simulink model "SRE_Integral"  (R2021a)
settings: Solver=VariableStepAuto  StartTime=0.0  StopTime=20.0  RelTol=1e-3
values from neighbouring files (symbols this model uses):
  G = ss(Ad, Bd, Cd, Dd, Ts)    [controlador_RE.m]    (also in realim_estados_no_ff.m)
  K = acker(A_ext, B_ext, exp(Ts*p_C))    [controlador_RE.m]    (also in realim_estados_no_ff.m = [0.2533,   -0.0121, -116.5175,  -30])
  L_o = [ 0.0003  0.0002 ... (first row only)    [controlador_RE.m]
  Ts = 20e-3    (= 0.02)    [controlador_RE.m]    (also in realim_estados_no_ff.m)
undefined symbols (not defined in the file or in its folder): DiscIntNeverNeededParam
libraries: simulink x1
settings Model: Creator=mathe  LastModifiedBy=mathe

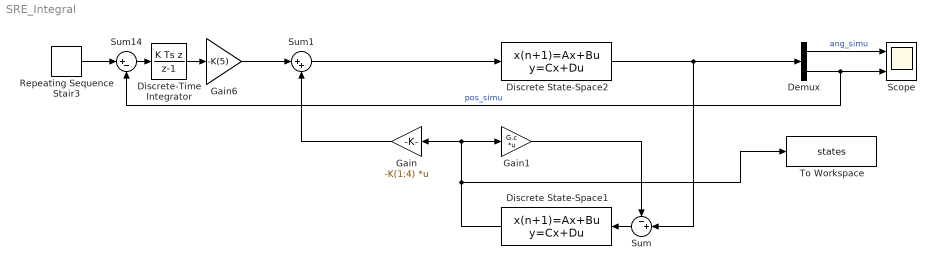
== system SRE_Integral ==
  Demux : Demux  Outputs=2
  Discrete State-Space1 : DiscreteStateSpace  A=G.a-G.b*K(1:4)  B=L_o  C=eye(4)  D=zeros(4,2)  InitialCondition=[0 0 0 0]  SampleTime=Ts
  Discrete State-Space2 : DiscreteStateSpace  A=G.a  B=G.b  C=G.c  D=zeros(2,1)  InitialCondition=[0 0 0 0]  SampleTime=Ts
  Discrete-Time Integrator : DiscreteIntegrator  IntegratorMethod=Integration: Backward Euler  SampleTime=-1  ICPrevOutput=DiscIntNeverNeededParam  ICPrevScaledInput=DiscIntNeverNeededParam
  Gain : Gain  Gain=-K(1:4)  Multiplication=Matrix(K*u)
  Gain1 : Gain  Gain=G.c  Multiplication=Matrix(K*u)
  Gain6 : Gain  Gain=-K(5)
  Repeating Sequence Stair3 : simulink/Sources/Repeating Sequence Stair  OutValues=[0 0.1 -.10].'  tsamp=5  OutMin=[]  OutMax=[]  OutDataTypeStr=double  OutputDataTypeScalingMode=double  OutDataType=fixdt(0,8)  ConRadixGroup=Best Precision: Vector-wise  OutScaling=2^-12
  Scope : Scope  NumInputPorts=2
  Sum : Sum  Inputs=-+|
  Sum1 : Sum  Inputs=|++
  Sum14 : Sum  Inputs=|+-
  To Workspace : ToWorkspace  VariableName=states  SampleTime=-1
      settings: Save2DSignal=2-D array (concatenate along first dimension)
  wires:
  Discrete State-Space1/1 -> To Workspace/1, Gain1/1, Gain/1
  Discrete State-Space2/1 -> Sum/2, Demux/1
  Demux/1 -> Scope/1  "ang_simu"
  Demux/2 -> Sum14/2, Scope/2  "pos_simu"
  Sum/1 -> Discrete State-Space1/1
  Gain1/1 -> Sum/1
  Gain/1 -> Sum1/2
  Sum1/1 -> Discrete State-Space2/1
  Gain6/1 -> Sum1/1
  Discrete-Time Integrator/1 -> Gain6/1
  Sum14/1 -> Discrete-Time Integrator/1
  Repeating Sequence Stair3/1 -> Sum14/1
